simulink model "Manimtim_Problem5"  (R2023b)
settings: Solver=VariableStepAuto  StartTime=0.0  StopTime=10.0  RelTol=1e-3
values from neighbouring files (symbols this model uses):
  G_den5 = [1 2 3 4 5 6 7 1]    [Manimtim_Problem5and6.m]
  G_num5 = [8 7 6 5 4 3 2]    [Manimtim_Problem5and6.m]
settings Model: Creator=John Kenneth  LastModifiedBy=John Kenneth

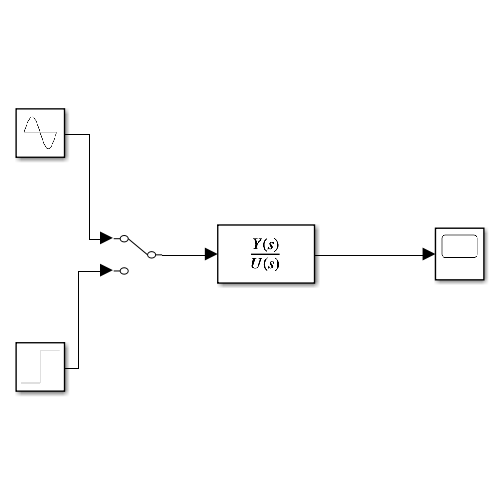
[thumbnail: Simulink's stored preview of the top-level diagram]
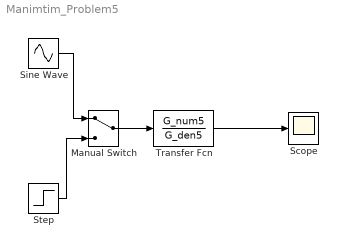
== system Manimtim_Problem5 ==
  Manual Switch : ManualSwitch
  Scope : Scope
  Sine Wave : Sin  SampleTime=0
  Step : Step  Time=0  SampleTime=0
  Transfer Fcn : TransferFcn  Numerator=G_num5  Denominator=G_den5
  wires:
  Sine Wave/1 -> Manual Switch/1
  Step/1 -> Manual Switch/2
  Manual Switch/1 -> Transfer Fcn/1
  Transfer Fcn/1 -> Scope/1
